simulink model "qp_torq_allocator"  (R2024b)
settings: Solver=FixedStepAuto  StartTime=0.0  StopTime=10.0  RelTol=1e-3
undefined symbols (not defined in the file): DiscIntNeverNeededParam
settings Model: Creator=lukec  LastModifiedBy=lukec
settings OptimizationCC: DefaultParameterBehavior=Inlined  EnhancedBackFolding=on  PassReuseOutputArgsAs=Individual arguments  ZeroExternalMemoryAtStartup=off  ZeroInternalMemoryAtStartup=off  OptimizeBlockOrder=speed  DifferentSizesBufferReuse=on  OptimizationCustomize=off  EfficientTunableParamExpr=on
settings DebuggingCC: ParameterTunabilityLossMsg=error
settings HardwareCC: ProdBitPerPointer=32  ProdBitPerSizeT=32  ProdBitPerPtrDiffT=32  ProdLargestAtomicInteger=Long  ProdLargestAtomicFloat=Double  ProdWordSize=32  ProdHWDeviceType=ARM Compatible->ARM Cortex-M
settings SFSimCC: MATLABDynamicMemAlloc=off
settings RTWCC: Description=Embedded Coder  SystemTargetFile=ert.tlc  GenCodeOnly=on  PackageGeneratedCodeAndArtifacts=on  TemplateMakefile=ert_default_tmf  Toolchain=CMake  TargetLang=C++  HalideCodeGeneration=on
settings CodeAppCC: ForceParamTrailComments=on  IgnoreCustomStorageClasses=off  MaxIdLength=255  OperatorAnnotations=on  SimulinkDataObjDesc=on  SFDataObjDesc=on  InsertBlockDesc=on
settings ERTTargetCC: TargetLangStandard=C++17 (ISO)  CodeInterfacePackaging=C++ class  RootIOFormat=Structure reference  ERTCustomFileTemplate=example_file_process.tlc  ArrayContainerType=std::array

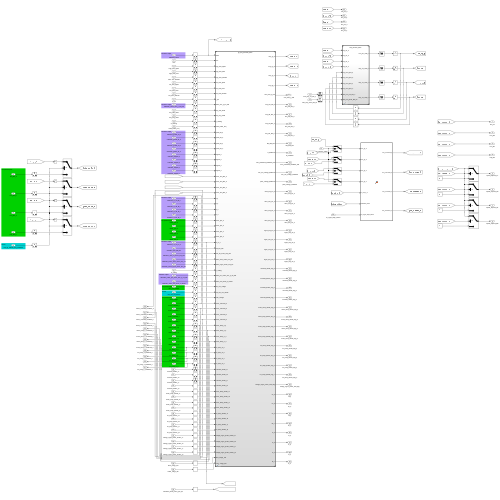
[thumbnail: Simulink's stored preview of the top-level diagram]
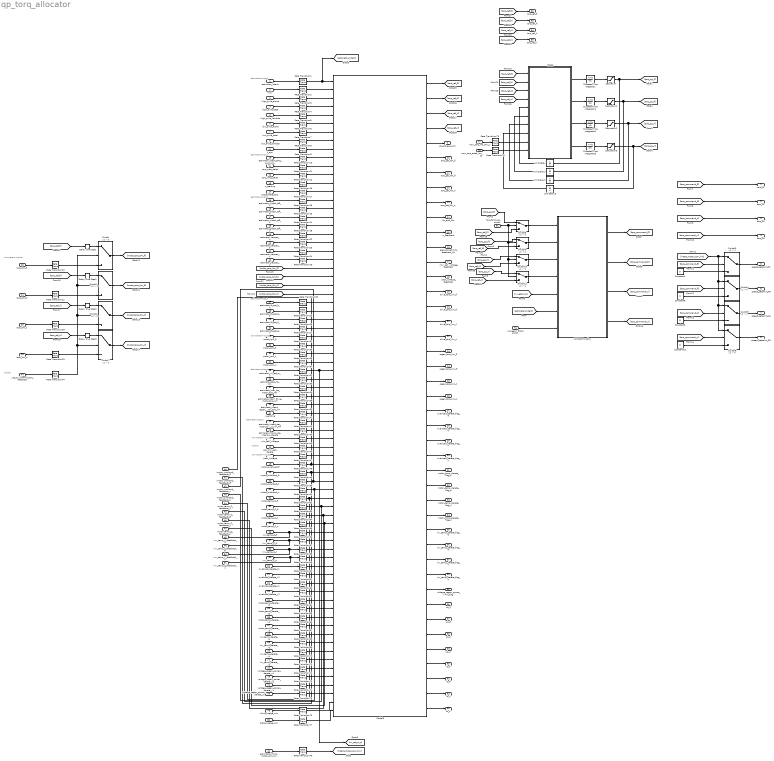
== system qp_torq_allocator ==
  note: non-param-inputs
  note: estimator-output
  note: estimator-output
  note: non-param-inputs
  note: estimator-output
  note: estimator-output
  note: estimator-output
  note: estimator-output
  note: is-bool
  note: non-param-inputs
  note: is-bool
  note: non-param-inputs
  estimator_intent : Inport
  mux : Inport  Port=2
  high_axle_alpha : Inport  Port=3
  high_axle_beta : Inport  Port=4
  high_axle_lambda : Inport  Port=5
  low_axle_alpha : Inport  Port=6
  low_axle_beta : Inport  Port=7
  low_axle_lambda : Inport  Port=8
  k_opt : Inport  Port=9
  estimator_intent_elec_p_lim_kW : Inport  Port=10
  torq_side_delta : Inport  Port=11
  torq_long_delta : Inport  Port=12
  w_starting : Inport  Port=13
  coast_brake_torq : Inport  Port=14
  estimator_global_eff_fl : Inport  Port=15
  estimator_global_eff_fr : Inport  Port=16
  estimator_global_eff_rl : Inport  Port=17
  estimator_global_eff_rr : Inport  Port=18
  estimator_kappas_fl : Inport  Port=19
  estimator_kappas_fr : Inport  Port=20
  estimator_kappas_rl : Inport  Port=21
  estimator_kappas_rr : Inport  Port=22
  torq_Nm_fl : Inport  Port=23
  torq_Nm_fr : Inport  Port=24
  torq_Nm_rl : Inport  Port=25
  torq_Nm_rr : Inport  Port=26
  estimator_fz_est_N_fl : Inport  Port=27
  estimator_fz_est_N_fr : Inport  Port=28
  estimator_fz_est_N_rl : Inport  Port=29
  estimator_fz_est_N_rr : Inport  Port=30
  motor_rpm_fl : Inport  Port=31
  motor_rpm_fr : Inport  Port=32
  motor_rpm_rl : Inport  Port=33
  motor_rpm_rr : Inport  Port=34
  estimator_vx_est_m_s : Inport  Port=35
  estimator_des_Mz_Nm : Inport  Port=36
  estimator_max_tot_motor_torq_Nm : Inport  Port=37
  estimator_intent_drive_motor_torq_lim : Inport  Port=38
  estimator_intent_regen_motor_torq_lim : Inport  Port=39
  estimator_intent_motor_rpm_lim : Inport  Port=40
  w_ending : Inport  Port=41
  estimator_intent_per_motor_elec_p_lim_kW : Inport  Port=42
  estimator_intent_use_intent_w_derate : Inport  Port=43
  use_qp_internal_torq_feedback : Inport  Port=44  OutDataTypeStr=boolean
  min_cell_voltage : Inport  Port=45
  use_min_cell_derate : Inport  Port=46  OutDataTypeStr=boolean
  pack_voltage : Inport  Port=47
  motor_overload_fl : Inport  Port=48
  motor_overload_fr : Inport  Port=49
  motor_overload_rl : Inport  Port=50
  motor_overload_rr : Inport  Port=51
  motor_temp_C_fl : Inport  Port=52
  motor_temp_C_fr : Inport  Port=53
  motor_temp_C_rl : Inport  Port=54
  motor_temp_C_rr : Inport  Port=55
  inv_temp_C_fl : Inport  Port=56
  inv_temp_C_fr : Inport  Port=57
  inv_temp_C_rl : Inport  Port=58
  inv_temp_C_rr : Inport  Port=59
  overload_derate_x1 : Inport  Port=60
  overload_derate_x2 : Inport  Port=61
  overload_derate_y1 : Inport  Port=62
  overload_derate_y2 : Inport  Port=63
  motor_temp_derate_x1 : Inport  Port=64
  motor_temp_derate_x2 : Inport  Port=65
  motor_temp_derate_y1 : Inport  Port=66
  motor_temp_derate_y2 : Inport  Port=67
  inv_temp_derate_x1 : Inport  Port=68
  inv_temp_derate_x2 : Inport  Port=69
  inv_temp_derate_y1 : Inport  Port=70
  inv_temp_derate_y2 : Inport  Port=71
  voltage_regen_power_derate_x1 : Inport  Port=72
  voltage_regen_power_derate_x2 : Inport  Port=73
  voltage_regen_power_derate_y1 : Inport  Port=74
  voltage_regen_power_derate_y2 : Inport  Port=75
  no_regen_5kph_switch : Inport  Port=76
  max_torq_vel_Nm_s : Inport  Port=77
  max_torq_accel_Nm_s2 : Inport  Port=78
  drive_usage_min : Inport  Port=79
  brake_usage_min : Inport  Port=80
  torq_follower_switch : Inport  Port=81
  Constant{4,6,8,10} (4 alike) : Constant  Value=0
  Delay One Step{,1..3} (4 alike) : Delay  DelayLength=1  SampleTime=0.004
  Discrete-Time Integrator{,1..3} (4 alike) : DiscreteIntegrator  SampleTime=0.004  ICPrevOutput=DiscIntNeverNeededParam  ICPrevScaledInput=DiscIntNeverNeededParam
  MATLAB Function : MATLAB Function  TreatAsAtomicUnit=on
  Model : ModelReference  ModelNameDialog=torq_follower_base.slx  SimulationMode=Normal  ModelReferenceVersion=1.6
      settings: PortSchema="{\"entries\":[{\"content\":{\"sides\":[{\"content\":{\"connectorIds\":[\"In1\",\"In3\",\"In5\",\"In7\",\"In2\",\"In4\",\"In6\",\"In8\",\"In9\",\"In10\"]},\"type\":\"ConnectorPlacement.EquallySpacedRectSide\",\"uuid\":\"f7d43a37-e4d7-4993-b7a1-7ee429905a8f\"},{\"content\":{\"connectorIds\":[\"Out1\",\"Out2\",\"Out3\",\"Out4\"],\"side\":\"RIGHT\"},\"type\":\"ConnectorPlacement.EquallySpacedRectSide\",\"uuid\":\"9ad1dd80-ab4f-41e1-9a6a-44c5d0d1936b\"},{\"content\":{\"side\":\"TOP\"},\"type\":\"ConnectorPlacement.EquallySpacedRectSide\",\"uuid\":\"1b048456-4925-4e4c-9a8a-1322b05dc2e7\"}]},\"type\":\"ConnectorPlacement.EquallySpacedConnector\",\"uuid\":\"7c415d82-e473-430f-8b80-0cc1ef57b436\"}],\"packageUris\":[\"http://schema.mathworks.com/mf0/Connector/R2020b\"],\"version\":\"1.0\"}"
  Model5 : ModelReference  ModelNameDialog=qp_torq_allocator_base.slx  SimulationMode=Normal  ModelReferenceVersion=1.43
  Rate Transition{1..79} (79 alike) : RateTransition  OutPortSampleTime=0.004
  Saturation{,1..3} (4 alike) : Saturate  UpperLimit=21  LowerLimit=-21
  Switch{,1..11} (12 alike) : Switch  Criteria=u2 > Threshold  SaturateOnIntegerOverflow=off  InputSameDT=off
  Unit Delay{,1..3} (4 alike) : UnitDelay  SampleTime=0.004  HasFrameUpgradeWarning=on
  torq_FL : Outport
  torq_FR : Outport  Port=2
  torq_RL : Outport  Port=3
  torq_RR : Outport  Port=4
  speed_setpoint_FL : Outport  Port=5
  speed_setpoint_FR : Outport  Port=6
  speed_setpoint_RL : Outport  Port=7
  speed_setpoint_RR : Outport  Port=8
  elec_theo_p_kW : Outport  Port=9
  torq_sat_Nm_fl : Outport  Port=10
  torq_sat_Nm_fr : Outport  Port=11
  torq_sat_Nm_rl : Outport  Port=12
  torq_sat_Nm_rr : Outport  Port=13
  Mz_add_Nm : Outport  Port=14
  w_feedback : Outport  Port=15
  elec_powerlimit_feedback_kW : Outport  Port=16
  min_cell_voltage_feedback : Outport  Port=17
  pack_voltage_feedback : Outport  Port=18
  drive_torq_lim_fl : Outport  Port=19
  drive_torq_lim_fr : Outport  Port=20
  drive_torq_lim_rl : Outport  Port=21
  drive_torq_lim_rr : Outport  Port=22
  regen_torq_lim_fl : Outport  Port=23
  regen_torq_lim_fr : Outport  Port=24
  regen_torq_lim_rl : Outport  Port=25
  regen_torq_lim_rr : Outport  Port=26
  overload_derate_flag_fl : Outport  Port=27
  overload_derate_flag_fr : Outport  Port=28
  overload_derate_flag_rl : Outport  Port=29
  overload_derate_flag_rr : Outport  Port=30
  motor_temp_derate_flag_fl : Outport  Port=31
  motor_temp_derate_flag_fr : Outport  Port=32
  motor_temp_derate_flag_rl : Outport  Port=33
  motor_temp_derate_flag_rr : Outport  Port=34
  inv_temp_derate_flag_fl : Outport  Port=35
  inv_temp_derate_flag_fr : Outport  Port=36
  inv_temp_derate_flag_rl : Outport  Port=37
  inv_temp_derate_flag_rr : Outport  Port=38
  voltage_regen_power_limit_flag : Outport  Port=39
  motor_overload_feedback_fl : Outport  Port=40
  motor_overload_feedback_fr : Outport  Port=41
  motor_overload_feedback_rl : Outport  Port=42
  motor_overload_feedback_rr : Outport  Port=43
  motor_temp_C_feedback_fl : Outport  Port=44
  motor_temp_C_feedback_fr : Outport  Port=45
  motor_temp_C_feedback_rl : Outport  Port=46
  motor_temp_C_feedback_rr : Outport  Port=47
  inv_temp_C_feedback_fl : Outport  Port=48
  inv_temp_C_feedback_fr : Outport  Port=49
  inv_temp_C_feedback_rl : Outport  Port=50
  inv_temp_C_feedback_rr : Outport  Port=51
  torq_ref_fl : Outport  Port=52
  torq_ref_fr : Outport  Port=53
  torq_ref_rl : Outport  Port=54
  torq_ref_rr : Outport  Port=55
  ub_fl : Outport  Port=56
  ub_fr : Outport  Port=57
  ub_rl : Outport  Port=58
  ub_rr : Outport  Port=59
  lb_fl : Outport  Port=60
  lb_fr : Outport  Port=61
  lb_rl : Outport  Port=62
  lb_rr : Outport  Port=63
  wires:
  estimator_intent/1 -> Rate Transition1/1
  mux/1 -> Rate Transition2/1
  high_axle_alpha/1 -> Rate Transition3/1
  high_axle_beta/1 -> Rate Transition4/1
  high_axle_lambda/1 -> Rate Transition5/1
  low_axle_alpha/1 -> Rate Transition6/1
  low_axle_beta/1 -> Rate Transition7/1
  low_axle_lambda/1 -> Rate Transition8/1
  k_opt/1 -> Rate Transition9/1
  estimator_intent_elec_p_lim_kW/1 -> Rate Transition10/1
  torq_side_delta/1 -> Rate Transition11/1
  torq_long_delta/1 -> Rate Transition12/1
  w_starting/1 -> Rate Transition16/1
  coast_brake_torq/1 -> Rate Transition17/1
  estimator_global_eff_fl/1 -> Rate Transition18/1
  estimator_global_eff_fr/1 -> Rate Transition13/1
  estimator_global_eff_rl/1 -> Rate Transition14/1
  estimator_global_eff_rr/1 -> Rate Transition15/1
  estimator_kappas_fl/1 -> Rate Transition22/1
  estimator_kappas_fr/1 -> Rate Transition23/1
  estimator_kappas_rl/1 -> Rate Transition24/1
  estimator_kappas_rr/1 -> Rate Transition19/1
  torq_Nm_fl/1 -> Rate Transition20/1
  torq_Nm_fr/1 -> Rate Transition21/1
  torq_Nm_rl/1 -> Rate Transition28/1
  torq_Nm_rr/1 -> Rate Transition29/1
  estimator_fz_est_N_fl/1 -> Rate Transition30/1
  estimator_fz_est_N_fr/1 -> Rate Transition25/1
  estimator_fz_est_N_rl/1 -> Rate Transition26/1
  estimator_fz_est_N_rr/1 -> Rate Transition27/1
  motor_rpm_fl/1 -> Rate Transition31/1
  motor_rpm_fr/1 -> Rate Transition35/1
  motor_rpm_rl/1 -> Rate Transition36/1
  motor_rpm_rr/1 -> Rate Transition37/1
  estimator_vx_est_m_s/1 -> Rate Transition32/1
  estimator_des_Mz_Nm/1 -> Rate Transition33/1
  estimator_max_tot_motor_torq_Nm/1 -> Rate Transition34/1
  estimator_intent_drive_motor_torq_lim/1 -> Rate Transition38/1
  estimator_intent_regen_motor_torq_lim/1 -> Rate Transition39/1
  Rate Transition1/1 -> [estimator_intent], Model5/1
  Rate Transition2/1 -> Model5/2
  Rate Transition3/1 -> Model5/3
  Rate Transition6/1 -> Model5/6
  Rate Transition5/1 -> Model5/5
  Rate Transition4/1 -> Model5/4
  Rate Transition8/1 -> Model5/8
  Rate Transition10/1 -> Model5/10
  Rate Transition11/1 -> Model5/11
  Rate Transition9/1 -> Model5/9
  Rate Transition12/1 -> Model5/12
  Rate Transition7/1 -> Model5/7
  Rate Transition14/1 -> Model5/17
  Rate Transition15/1 -> Model5/18
  Rate Transition16/1 -> Model5/13
  Rate Transition17/1 -> Model5/14
  Rate Transition13/1 -> Model5/16
  Rate Transition18/1 -> Model5/15
  Rate Transition19/1 -> Model5/22
  Rate Transition24/1 -> Model5/21
  Rate Transition22/1 -> Model5/19
  Rate Transition23/1 -> Model5/20
  Rate Transition26/1 -> Model5/29
  Rate Transition27/1 -> Model5/30
  Rate Transition30/1 -> Model5/27
  Rate Transition25/1 -> Model5/28
  Rate Transition31/1 -> Model5/31
  Rate Transition32/1 -> [vx_est_m_s], Model5/35
  Rate Transition33/1 -> Model5/36
  Rate Transition34/1 -> Model5/37
  Rate Transition35/1 -> Model5/32
  Rate Transition36/1 -> Model5/33
  Rate Transition37/1 -> Model5/34
  Rate Transition39/1 -> Model5/39
  Rate Transition38/1 -> Model5/38
  estimator_intent_motor_rpm_lim/1 -> Rate Transition40/1
  Rate Transition40/1 -> [intent_motor_rpm_lim]
  Constant8/1 -> Switch5/3
  Switch4/1 -> speed_setpoint_FR/1
  Switch3/1 -> speed_setpoint_FL/1
  [torq_command_fr] -> Switch4/2
  [intent_motor_rpm_lim] -> Switch6/1, Switch5/1, Switch4/1, Switch3/1
  Switch6/1 -> speed_setpoint_RR/1
  [torq_command_rr] -> Switch6/2
  Constant4/1 -> Switch3/3
  [torq_command_rl] -> Switch5/2
  Constant6/1 -> Switch4/3
  Constant10/1 -> Switch6/3
  [torq_command_fl] -> Switch3/2
  Switch5/1 -> speed_setpoint_RL/1
  Model5/5 -> elec_theo_p_kW/1
  Model5/6 -> torq_sat_Nm_fl/1
  Model5/7 -> torq_sat_Nm_fr/1
  Model5/8 -> torq_sat_Nm_rl/1
  Model5/9 -> torq_sat_Nm_rr/1
  Model5/10 -> Mz_add_Nm/1
  [vx_est_m_s] -> MATLAB Function/5(vx_est_m_s)
  [estimator_intent] -> MATLAB Function/6(estimator_intent)
  MATLAB Function/1(torq_command_fl) -> [torq_command_fl]
  MATLAB Function/2(torq_command_fr) -> [torq_command_fr]
  MATLAB Function/3(torq_command_rl) -> [torq_command_rl]
  MATLAB Function/4(torq_command_rr) -> [torq_command_rr]
  [torq_command_fl] -> torq_FL/1
  [torq_command_fr] -> torq_FR/1
  [torq_command_rl] -> torq_RL/1
  [torq_command_rr] -> torq_RR/1
  Model5/11 -> w_feedback/1
  w_ending/1 -> Rate Transition41/1
  Rate Transition42/1 -> Model5/41
  Rate Transition41/1 -> Model5/40
  estimator_intent_per_motor_elec_p_lim_kW/1 -> Rate Transition42/1
  estimator_intent_use_intent_w_derate/1 -> Rate Transition43/1
  Rate Transition43/1 -> Model5/42
  use_qp_internal_torq_feedback/1 -> Rate Transition44/1
  Rate Transition44/1 -> Switch2/2, Switch/2, Switch1/2, Switch7/2
  Rate Transition20/1 -> Switch/3
  [torq_ref_fl] -> Delay One Step/1
  Delay One Step/1 -> Switch/1
  Delay One Step1/1 -> Switch1/1
  Delay One Step2/1 -> Switch2/1
  Delay One Step3/1 -> Switch7/1
  [torq_ref_fr] -> Delay One Step1/1
  [torq_ref_rl] -> Delay One Step2/1
  [torq_ref_rr] -> Delay One Step3/1
  Rate Transition21/1 -> Switch1/3
  Rate Transition28/1 -> Switch2/3
  Rate Transition29/1 -> Switch7/3
  Model5/12 -> elec_powerlimit_feedback_kW/1
  min_cell_voltage/1 -> Rate Transition45/1
  use_min_cell_derate/1 -> Rate Transition46/1
  Switch/1 -> [motor_torq_Nm_fl]
  Switch1/1 -> [motor_torq_Nm_fr]
  Switch2/1 -> [motor_torq_Nm_rl]
  Switch7/1 -> [motor_torq_Nm_rr]
  [motor_torq_Nm_fl] -> Model5/23
  [motor_torq_Nm_fr] -> Model5/24
  [motor_torq_Nm_rr] -> Model5/26
  [motor_torq_Nm_rl] -> Model5/25
  pack_voltage/1 -> Rate Transition47/1
  Model5/14 -> pack_voltage_feedback/1
  motor_overload_fl/1 -> Rate Transition48/1
  motor_overload_fr/1 -> Rate Transition49/1
  motor_overload_rl/1 -> Rate Transition50/1
  motor_overload_rr/1 -> Rate Transition51/1
  motor_temp_C_fl/1 -> Rate Transition52/1
  motor_temp_C_fr/1 -> Rate Transition53/1
  motor_temp_C_rl/1 -> Rate Transition54/1
  motor_temp_C_rr/1 -> Rate Transition55/1
  inv_temp_C_fl/1 -> inv_temp_C_feedback_fl/1, Rate Transition56/1
  inv_temp_C_fr/1 -> inv_temp_C_feedback_fr/1, Rate Transition57/1
  inv_temp_C_rl/1 -> inv_temp_C_feedback_rl/1, Rate Transition58/1
  inv_temp_C_rr/1 -> inv_temp_C_feedback_rr/1, Rate Transition59/1
  Rate Transition50/1 -> motor_overload_feedback_rl/1, Model5/48
  Rate Transition49/1 -> motor_overload_feedback_fr/1, Model5/47
  Rate Transition45/1 -> Model5/43
  Rate Transition47/1 -> Model5/45
  Rate Transition48/1 -> motor_overload_feedback_fl/1, Model5/46
  Rate Transition46/1 -> Model5/44
  Rate Transition52/1 -> motor_temp_C_feedback_fl/1, Model5/50
  Rate Transition53/1 -> motor_temp_C_feedback_fr/1, Model5/51
  Rate Transition55/1 -> motor_temp_C_feedback_rr/1, Model5/53
  Rate Transition54/1 -> motor_temp_C_feedback_rl/1, Model5/52
  Rate Transition56/1 -> Model5/54
  Rate Transition51/1 -> motor_overload_feedback_rr/1, Model5/49
  Rate Transition58/1 -> Model5/56
  Rate Transition59/1 -> Model5/57
  Rate Transition57/1 -> Model5/55
  overload_derate_x1/1 -> Rate Transition60/1
  overload_derate_x2/1 -> Rate Transition61/1
  overload_derate_y1/1 -> Rate Transition62/1
  overload_derate_y2/1 -> Rate Transition63/1
  motor_temp_derate_x1/1 -> Rate Transition64/1
  motor_temp_derate_x2/1 -> Rate Transition65/1
  motor_temp_derate_y1/1 -> Rate Transition66/1
  motor_temp_derate_y2/1 -> Rate Transition67/1
  inv_temp_derate_x1/1 -> Rate Transition68/1
  inv_temp_derate_x2/1 -> Rate Transition69/1
  inv_temp_derate_y1/1 -> Rate Transition70/1
  inv_temp_derate_y2/1 -> Rate Transition71/1
  Rate Transition67/1 -> Model5/65
  Rate Transition63/1 -> Model5/61
  Rate Transition65/1 -> Model5/63
  Rate Transition64/1 -> Model5/62
  Rate Transition61/1 -> Model5/59
  Rate Transition66/1 -> Model5/64
  Rate Transition68/1 -> Model5/66
  Rate Transition69/1 -> Model5/67
  Rate Transition70/1 -> Model5/68
  Rate Transition71/1 -> Model5/69
  Rate Transition62/1 -> Model5/60
  Rate Transition60/1 -> Model5/58
  voltage_regen_power_derate_x1/1 -> Rate Transition72/1
  voltage_regen_power_derate_x2/1 -> Rate Transition73/1
  voltage_regen_power_derate_y1/1 -> Rate Transition74/1
  voltage_regen_power_derate_y2/1 -> Rate Transition75/1
  Rate Transition72/1 -> Model5/70
  Rate Transition73/1 -> Model5/71
  Rate Transition74/1 -> Model5/72
  Rate Transition75/1 -> Model5/73
  Model5/13 -> min_cell_voltage_feedback/1
  Model5/15 -> drive_torq_lim_fl/1
  Model5/16 -> drive_torq_lim_fr/1
  Model5/17 -> drive_torq_lim_rl/1
  Model5/18 -> drive_torq_lim_rr/1
  Model5/19 -> regen_torq_lim_fl/1
  Model5/20 -> regen_torq_lim_fr/1
  Model5/21 -> regen_torq_lim_rl/1
  Model5/22 -> regen_torq_lim_rr/1
  Model5/23 -> overload_derate_flag_fl/1
  Model5/24 -> overload_derate_flag_fr/1
  Model5/25 -> overload_derate_flag_rl/1
  Model5/26 -> overload_derate_flag_rr/1
  Model5/27 -> motor_temp_derate_flag_fl/1
  Model5/28 -> motor_temp_derate_flag_fr/1
  Model5/29 -> motor_temp_derate_flag_rl/1
  Model5/30 -> motor_temp_derate_flag_rr/1
  Model5/31 -> inv_temp_derate_flag_fl/1
  Model5/32 -> inv_temp_derate_flag_fr/1
  Model5/33 -> inv_temp_derate_flag_rl/1
  Model5/34 -> inv_temp_derate_flag_rr/1
  Model5/35 -> voltage_regen_power_limit_flag/1
  no_regen_5kph_switch/1 -> MATLAB Function/7(no_regen_5kph_switch)
  Model5/1 -> [torq_ref_fl]
  [torq_ref_fl] -> Model/1
  Model/1 -> Discrete-Time Integrator/1
  Discrete-Time Integrator/1 -> Saturation/1
  Saturation/1 -> [torq_qp_fl], Unit Delay/1
  Unit Delay/1 -> Model/2
  Model5/2 -> [torq_ref_fr]
  Model5/3 -> [torq_ref_rl]
  Model5/4 -> [torq_ref_rr]
  [torq_ref_fr] -> Model/3
  [torq_ref_rl] -> Model/5
  [torq_ref_rr] -> Model/7
  Discrete-Time Integrator1/1 -> Saturation1/1
  Discrete-Time Integrator2/1 -> Saturation2/1
  Discrete-Time Integrator3/1 -> Saturation3/1
  Model/2 -> Discrete-Time Integrator1/1
  Model/3 -> Discrete-Time Integrator2/1
  Model/4 -> Discrete-Time Integrator3/1
  Saturation1/1 -> Unit Delay1/1, [torq_qp_fr]
  Saturation2/1 -> Unit Delay2/1, [torq_qp_rl]
  Saturation3/1 -> Unit Delay3/1, [torq_qp_rr]
  Unit Delay1/1 -> Model/4
  Unit Delay2/1 -> Model/6
  Unit Delay3/1 -> Model/8
  [torq_ref_fl] -> torq_ref_fl/1
  [torq_ref_fr] -> torq_ref_fr/1
  [torq_ref_rl] -> torq_ref_rl/1
  [torq_ref_rr] -> torq_ref_rr/1
  max_torq_vel_Nm_s/1 -> Rate Transition78/1
  max_torq_accel_Nm_s2/1 -> Rate Transition79/1
  drive_usage_min/1 -> Rate Transition76/1
  Rate Transition76/1 -> Model5/74
  brake_usage_min/1 -> Rate Transition77/1
  Rate Transition77/1 -> Model5/75
  Model5/36 -> ub_fl/1
  Model5/37 -> ub_fr/1
  Model5/38 -> ub_rl/1
  Model5/39 -> ub_rr/1
  Model5/40 -> lb_fl/1
  Model5/41 -> lb_fr/1
  Model5/42 -> lb_rl/1
  Model5/43 -> lb_rr/1
  Rate Transition78/1 -> Model/9
  Rate Transition79/1 -> Model/10
  torq_follower_switch/1 -> Switch10/2, Switch11/2, Switch9/2, Switch8/2
  [torq_qp_fl] -> Switch8/1
  Switch8/1 -> MATLAB Function/1(torq_qp_fl)
  [torq_ref_fl] -> Switch8/3
  Switch9/1 -> MATLAB Function/2(torq_qp_fr)
  Switch10/1 -> MATLAB Function/3(torq_qp_rl)
  Switch11/1 -> MATLAB Function/4(torq_qp_rr)
  [torq_qp_fr] -> Switch9/1
  [torq_qp_rl] -> Switch10/1
  [torq_qp_rr] -> Switch11/1
  [torq_ref_rr] -> Switch11/3
  [torq_ref_rl] -> Switch10/3
  [torq_ref_fr] -> Switch9/3

== matlab function qp_torq_allocator/MATLAB Function ==
  data: torq_qp_fl input; torq_command_fl output; torq_qp_fr input; torq_qp_rl input; torq_qp_rr input; vx_est_m_s input; torq_command_fr output; torq_command_rl output; torq_command_rr output; estimator_intent input; no_regen_5kph_switch input
function [torq_command_fl, torq_command_fr, torq_command_rl, torq_command_rr] = fcn(torq_qp_fl, torq_qp_fr, torq_qp_rl, torq_qp_rr, vx_est_m_s, estimator_intent, no_regen_5kph_switch)

    switch no_regen_5kph_switch
        case 1
        case 0
        otherwise
            no_regen_5kph_switch = 1;
    end

    if no_regen_5kph_switch == 0
        torq_command_fl = torq_qp_fl;
        torq_command_fr = torq_qp_fr;
        torq_command_rl = torq_qp_rl;
        torq_command_rr = torq_qp_rr;
    else

        regen_derate_speed = 10/3.6;
        no_regen_speed = 5/3.6;
    
        if vx_est_m_s < no_regen_speed
            
            % speed under 5 KPH
    
            if estimator_intent < 0
    
                % Attempting to brake, cut regen
                torq_command_fl = 0;
                torq_command_fr = 0;
                torq_command_rl = 0;
                torq_command_rr = 0;
    
            else
    
                % passthrough
                torq_command_fl = torq_qp_fl;
                torq_command_fr = torq_qp_fr;
                torq_command_rl = torq_qp_rl;
                torq_command_rr = torq_qp_rr;
    
            end
    
        elseif vx_est_m_s < regen_derate_speed && vx_est_m_s > no_regen_speed
    
            % speed greater than 5 KPH and less than 10 KPH
    
            if estimator_intent < 0
    
                % Attempting to brake
                gain = interp1([no_regen_speed, regen_derate_speed], [0, 1], vx_est_m_s);
    
                torq_command_fl = torq_qp_fl * gain;
                torq_command_fr = torq_qp_fr * gain;
                torq_command_rl = torq_qp_rl * gain;
                torq_command_rr = torq_qp_rr * gain;
    
            else
    
                % passthrough
                torq_command_fl = torq_qp_fl;
                torq_command_fr = torq_qp_fr;
                torq_command_rl = torq_qp_rl;
                torq_command_rr = torq_qp_rr;
    
            end
    
        else
            
            % speed above 10 KPH
            torq_command_fl = torq_qp_fl;
            torq_command_fr = torq_qp_fr;
            torq_command_rl = torq_qp_rl;
            torq_command_rr = torq_qp_rr;
    
        end

    end
